simulink model "s2"  (R2024a)
settings: Solver=VariableStepAuto  StartTime=0.0  StopTime=50  MaxStep=1/128  RelTol=1e-3
settings Model: Creator=hj53889  LastModifiedBy=gm54508

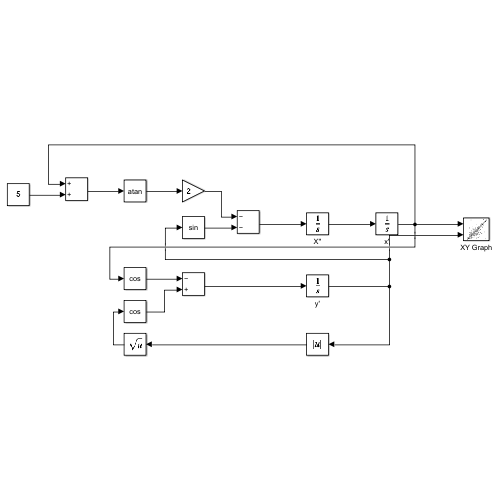
[thumbnail: Simulink's stored preview of the top-level diagram]
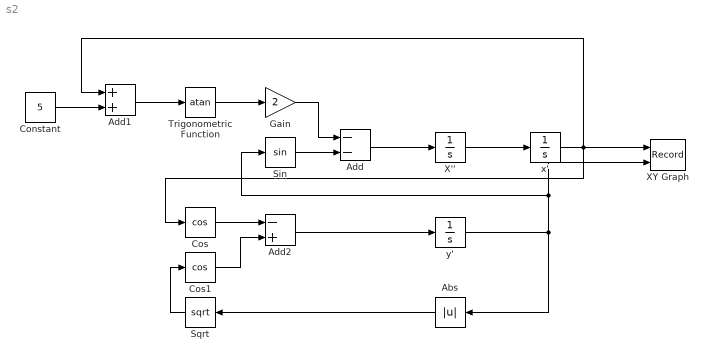
== system s2 ==
  Abs : Abs  SaturateOnIntegerOverflow=off
  Add : Sum  Inputs=--
  Add1 : Sum
  Add2 : Sum  Inputs=-+
  Constant : Constant  Value=5
  Cos : Trigonometry  Operator=cos
  Cos1 : Trigonometry  Operator=cos
  Gain : Gain  Gain=2
  Sin : Trigonometry
  Sqrt : Sqrt
  Trigonometric Function : Trigonometry  Operator=atan
  X'' : Integrator
  XY Graph : Record  FileSettingsInternal="{\"entries\":[{\"content\":{\"excelSettings\":{\"content\":{},\"type\":\"Streamout.ExcelSettings\"}},\"type\":\"Streamout.FileSettingStorage\",\"uuid\":\"\"}],\"packageUris\":[\"http:\\/\\/schema.mathworks.com\\/mf0\\/streamout_blocks\\/R2020a\"],\"version\":\"1.0\"}"  Layout=[1 1]  SignalsInternal="{\"entries\":[{\"content\":{\"signals\":[{\"content\":{\"blockPath\":[],\"dimensions\":[1],\"domain\":\"\",\"lineColor\":\"#a2142f\",\"plots\":[ 1 ],\"port\":1,\"sid\":[\"\"],\"signalID\":1,\"signalName\":\"x'\"},\"type\":\"RecordBlkView.Signal\",\"uuid\":\"\"},{\"content\":{\"blockPath\":[],\"dimensions\":[1],\"domain\":\"\",\"lineColor\":\"#139fff\",\"plots\":[ 1 ],\"port\":2,\"sid\":[\"\"],\"signalID\":2,\"signalName\":\"y'\"},\"type\":\"RecordBlkView.Signal\",\"uuid\":\"\"}]},\"type\":\"RecordBlkView.InputSignals\",\"uuid\":\"\"}],\"packageUris\":[\"http:\\/\\/schema.mathworks.com\\/mf0\\/streamout_blocks\\/R2020a\"],\"version\":\"1.0\"}"  VisualizationBindings="{\"xyplotplugin\":{\"info\":[{\"series\":[{\"bindingParametersList\":[{\"parameter\":\"X-Axis\",\"signalID\":1,\"signalName\":\"x'\"},{\"parameter\":\"Y-Axis\",\"signalID\":2,\"signalName\":\"y'\"}],\"seriesID\":0}],\"subplotID\":1}]}}"  CompatibilityTag=XY
  x' : Integrator  InitialCondition=1
  y' : Integrator  InitialCondition=2
  wires:
  X''/1 -> x'/1
  Add/1 -> X''/1
  Constant/1 -> Add1/2
  x'/1 -> Add1/1, XY Graph/1, Cos/1
  Add1/1 -> Trigonometric Function/1
  y'/1 -> Abs/1, XY Graph/2, Sin/1
  Sin/1 -> Add/2
  Add2/1 -> y'/1
  Cos/1 -> Add2/1
  Cos1/1 -> Add2/2
  Sqrt/1 -> Cos1/1
  Abs/1 -> Sqrt/1
  Trigonometric Function/1 -> Gain/1
  Gain/1 -> Add/1
